simulink model "simulinkmdl"  (R2016b)
settings: Solver=FixedStepDiscrete  StartTime=0.0  StopTime=steps*ts  FixedStep=ts  RelTol=1e-3
values from neighbouring files (symbols this model uses):
  B = Bsys    [Plant10_NMPChzNMPTz.m]
  C = E1    [Plant10_NMPChzNMPTz.m]
  D0 = Dsys    [Plant10_NMPChzNMPTz.m]
  ts = 1    [PlantBuilderNMPConfigRCAC.m]
undefined symbols (not defined in the file or in its folder): A
settings Model: Creator=Nima  LastModifiedBy=Nima
settings RTWCC: Toolchain=MinGW64 v4.x | gmake (64-bit Windows)  TargetLang=C++
settings GRTTargetCC: TargetLangStandard=C++03 (ISO)  MultiInstanceERTCode=on  CodeInterfacePackaging=C++ class

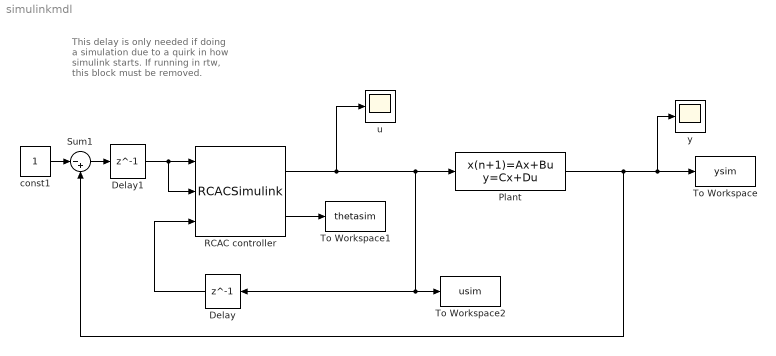
== system simulinkmdl ==
  note: This delay is only needed if doing a simulation due to a quirk in how simulink starts.
      | If running in rtw, this block must be removed.
  Delay : Delay  DelayLength=1  InitialCondition=0
  Delay1 : Delay  DelayLength=1  InitialCondition=0
  Plant : DiscreteStateSpace  A=A  B=B  C=C  D=D0  SampleTime=ts
  RCAC controller : S-Function  FunctionName=RCACSimulink  Parameters=ts, rcactype, mexFLAGS, mexFILT  SFunctionModules=RCAC RCACRLS  SFunctionDeploymentMode=off  EnableBusSupport=off
      mask Display:
      | port_label('input', 1, 'z')
      | port_label('input', 2, 'y')
      | port_label('input', 3, 'u')
      | port_label('output', 1, 'u')
      | port_label('output', 2, 'theta')
      | 
      | disp('RCAC')
  Sum1 : Sum  Inputs=|-+
  To Workspace : ToWorkspace  VariableName=ysim  SampleTime=-1
      settings: Save2DSignal=2-D array (concatenate along first dimension)
  To Workspace1 : ToWorkspace  VariableName=thetasim  SampleTime=-1
  To Workspace2 : ToWorkspace  VariableName=usim  SampleTime=-1
  const1 : Constant
  u : Scope
  y : Scope
  wires:
  Delay/1 -> RCAC controller/3
  const1/1 -> Sum1/1
  RCAC controller/2 -> To Workspace1/1
  Delay1/1 -> RCAC controller/2, RCAC controller/1
  Plant/1 -> Sum1/2, y/1, To Workspace/1
  Sum1/1 -> Delay1/1
  RCAC controller/1 -> Plant/1, Delay/1, To Workspace2/1, u/1
